simulink model "modelo_nioc_obs"  (R2023a)
settings: Solver=ode15s  StartTime=0.0  StopTime=100  RelTol=1e-3
InitFcn:
  | clc
  | clear
  | close all
  | parametros
  | gain_CL
  | calculo_observador_carro
  | calculo_observador_izaje
values from neighbouring files (symbols this model uses):
  At = [ 0, 1, 0, 0 ... (first row only)    [calculo_observador_carro.m]
  b_cx = 1e6    (= 1000000)    [parametros.m]
  b_cy = 1e7    (= 10000000)    [parametros.m]
  b_ha = -(J_hEq + (r_hd/(2*i_h))*m_l) * w_des_h*(1 + n_h + n_h^2) + b_hEq    [gain_CL.m]
  b_hb = 1e8    (= 100000000)    [parametros.m]
  b_hd = 8    [parametros.m]
  b_hm = 18    [parametros.m]
  b_t = 90    [parametros.m]
  b_ta = M_tEq*w_des_t*(1+n_t+n_t^2)-b_tEq    [gain_CL.m]
  b_tb = 5e6    (= 5000000)    [parametros.m]
  b_td = 1.8    [parametros.m]
  b_tm = 6    [parametros.m]
  b_tw = 3e3    (= 3000)    [parametros.m]
  b_wu = 150    [parametros.m]
  Bct = [ 0, 0 ... (first row only)    [calculo_observador_carro.m]
  Bdt = [ 0 ... (first row only)    [calculo_observador_carro.m]
  Ct = [ 1, 0, 0, 0 ]    [calculo_observador_carro.m]
  g = 9.80665    [parametros.m]
  H_c = 2.59    [parametros.m]
  i_h = 22    [parametros.m]
  i_t = 30    [parametros.m]
  J_hd_hEb = 3800    [parametros.m]
  J_hm_hb = 30    [parametros.m]
  J_td = 1200    [parametros.m]
  J_tm_tb = 7    [parametros.m]
  K_cy = 1.8e9    (= 1800000000)    [parametros.m]
  k_hsa = -(J_hEq + (r_hd/(2*i_h))*m_l) * w_des_h^2*(n_h + n_h^2 + n_h^3)    [gain_CL.m]
  k_hsia = -(J_hEq + (r_hd/(2*i_h))*m_l) * n_h^3 * w_des_h^3    [gain_CL.m]
  k_tsa = M_tEq*w_des_t^2*n_t*(1+n_t+n_t^2)    [gain_CL.m]
  k_tsia = M_tEq*w_des_t^3*n_t^3    [gain_CL.m]
  K_tw = 4.8e5    (= 480000)    [parametros.m]
  k_wu = 2.36e8    (= 236000000)    [parametros.m]
  l_h0 = (Y_t0-y_l0)    (= 38)    [parametros.m]
  Lt = place(At', Ct', polos_deseados)'    [calculo_observador_carro.m]
  M_cmax = 50000    [parametros.m]
  M_cmin = 2000    [parametros.m]
  m_l = M_s    (= 15000)    [parametros.m]
  M_s = 15000    [parametros.m]
  M_t = 30000    [parametros.m]
  M_tEq = i_t/r_td*(J_tm_tb+J_td/i_t^2)+r_td/i_t*(M_t+m_l)    (= 1250)    [parametros.m]
  r_hd = 0.75    [parametros.m]
  r_td = 0.50    (= 0.5)    [parametros.m]
  T_hbMax = 5e4    (= 50000)    [parametros.m]
  T_hEbMax = 1.1e6    (= 1100000)    [parametros.m]
  T_hmMax = 2e4    (= 20000)    [parametros.m]
  T_s = 0.001    [parametros.m]
  T_tbMax = 5e3    (= 5000)    [parametros.m]
  T_tmMax = 4e3    (= 4000)    [parametros.m]
  tau_tm = 1e-3    (= 0.001)    [parametros.m]
  theta_hm0 = -l_h0*i_h*2/r_hd    (= -2229.33333333)    [parametros.m]
  theta_tm0 = (x_t0)*i_t/r_td    (= -900)    [parametros.m]
  v_h_max_noload = 3    [parametros.m]
  v_lx0 = 0    [parametros.m]
  v_ly0 = 0    [parametros.m]
  v_t0 = 0    [parametros.m]
  v_t_max = 4    [parametros.m]
  W_c = ctrb(A, B_c(:,1))    [CyO_carro.m]    (also in CyO_izaje.m; parametros.m = 2.44)
  w_hm0 = 0    [parametros.m]
  w_hm_rated = v_h_max_load*2*i_h/r_hd    (= 88)    [parametros.m]
  w_tm0 = (v_t0)*i_t/r_td    (= 0)    [parametros.m]
  x_l0 = x_t0    (= -15)    [parametros.m]
  x_lidar_offset = 3.0    (= 3)    [parametros.m]
  x_t0 = -15    [parametros.m]
  x_t_max = 50    [parametros.m]
  x_t_maxE = x_t_max+0.5    (= 50.5)    [parametros.m]
  x_t_min = -30    [parametros.m]
  x_t_minE = x_t_min-0.5    (= -30.5)    [parametros.m]
  y_h_max = 40    [parametros.m]
  y_h_maxE = y_h_max+0.5    (= 40.5)    [parametros.m]
  y_h_min = -20    [parametros.m]
  y_h_minE = y_h_min-0.5    (= -20.5)    [parametros.m]
  y_l0 = 7    [parametros.m]
  Y_sb = 5.0    (= 5)    [parametros.m]
  Y_t0 = 45    [parametros.m]
undefined symbols (not defined in the file or in its folder): Lh
libraries: dspsigops x1, simulink x1
settings Model: Creator=Usuario  LastModifiedBy=nsorr

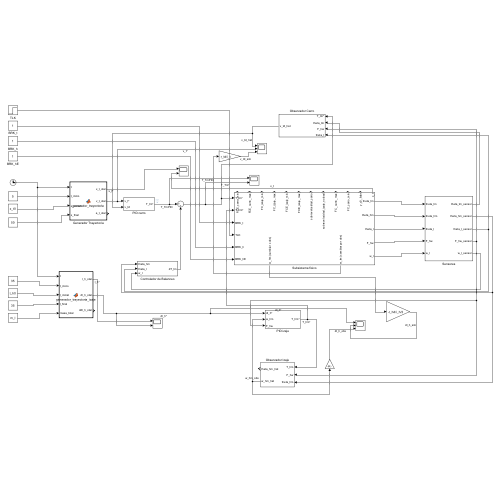
[thumbnail: Simulink's stored preview of the top-level diagram]
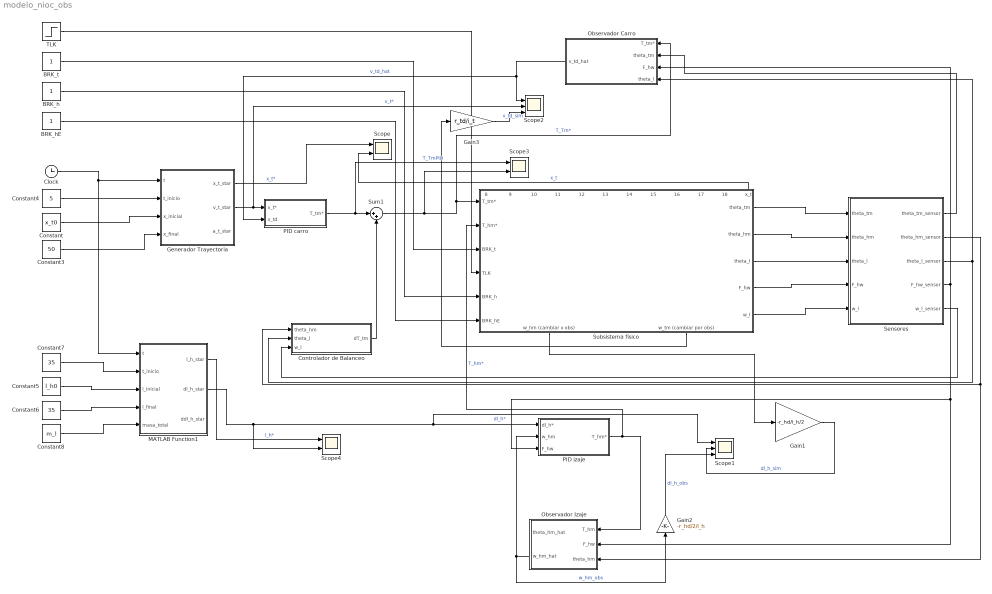
== system modelo_nioc_obs ==
  BRK_h : Constant
  BRK_hE : Constant
  BRK_t : Constant
  Clock : Clock
  Constant : Constant  Value=x_t0
  Constant3 : Constant  Value=50
  Constant4 : Constant  Value=5
  Constant5 : Constant  Value=l_h0
  Constant6 : Constant  Value=35
  Constant7 : Constant  Value=35
  Constant8 : Constant  Value=m_l
  Controlador de Balanceo : Subsystem
  Gain1 : Gain  Gain=-r_hd/i_h/2
  Gain2 : Gain  Gain=-r_hd/2/i_h
  Gain3 : Gain  Gain=r_td/i_t
  Generador Trayectoria : MATLAB Function  TreatAsAtomicUnit=on
  MATLAB Function1 : MATLAB Function  TreatAsAtomicUnit=on
  Observador Carro : Subsystem
  Observador Izaje : Subsystem
  PID carro : Subsystem
  PID izaje : Subsystem
  Scope : Scope  NumInputPorts=2
  Scope1 : Scope  NumInputPorts=3
  Scope2 : Scope  NumInputPorts=3
  Scope3 : Scope  NumInputPorts=2
  Scope4 : Scope  NumInputPorts=2
  Sensores : Subsystem
  Subsistema físico : Subsystem
      settings: PortSchema="{\"entries\":[{\"content\":{\"sides\":[{\"content\":{\"connectorIds\":[\"In1\",\"In2\",\"In3\",\"In4\",\"In5\",\"In6\"]},\"type\":\"ConnectorPlacement.EquallySpacedRectSide\",\"uuid\":\"aa1cb789-2051-45a4-8cb8-6dd2078290cc\"},{\"content\":{\"connectorIds\":[\"Out1\",\"Out2\",\"Out3\",\"Out4\",\"Out5\"],\"side\":\"RIGHT\"},\"type\":\"ConnectorPlacement.EquallySpacedRectSide\",\"uuid\":\"7fe62279-dd3b-46db-ba9e-e4633dcea5c6\"},{\"content\":{\"connectorIds\":[\"Out8\",\"Out9\",\"Out10\",\"Out11\",\"Out12\",\"Out13\",\"Out14\",\"Out15\",\"Out16\",\"Out17\",\"Out18\",\"Out19\"],\"side\":\"TOP\"},\"type\":\"ConnectorPlacement.EquallySpacedRectSide\",\"uuid\":\"a5663ea7-10d8-47d7-b8ed-8fbfb239b85a\"},{\"content\":{\"connectorIds\":[\"Out6\",\"Out7\"],\"side\":\"BOTTOM\"},\"type\":\"ConnectorPlacement.EquallySpacedRectSide\",\"uuid\":\"9ec9131f-7b2f-42d7-8a86-9462c3c282b3\"}]},\"type\":\"ConnectorPlacement.EquallySpacedConnector\",\"uuid\":\"e7df1a56-7803-4e0d-8bf9-081877eb8c08\"}],\"packageUris\":[\"http://schema.mathworks.com/mf0/Connector/R2020b\"],\"version\":\"1.0\"}"
  Sum1 : Sum  Inputs=|++
  TLK : Step  Time=5  SampleTime=0
  wires:
  Constant8/1 -> MATLAB Function1/5(masa_total)
  Generador Trayectoria/2(v_t_star) -> Scope2/2, PID carro/1(v_t*)  "v_t*"
  Constant7/1 -> MATLAB Function1/2(t_inicio)
  BRK_h/1 -> Subsistema físico/5(BRK_h)
  Constant6/1 -> MATLAB Function1/4(l_final)
  PID carro/1(T_tm*) -> Scope3/1, Sum1/1  "T_TmPID"
  BRK_t/1 -> Subsistema físico/3(BRK_t)
  Subsistema físico/2(theta_hm) -> Sensores/2(theta_hm)
  Constant4/1 -> Generador Trayectoria/2(t_inicio)
  Constant5/1 -> MATLAB Function1/3(l_inicial)
  MATLAB Function1/2(dl_h_star) -> Scope4/2, Scope1/1, PID izaje/1(dl_h*)  "dl_h*"
  BRK_hE/1 -> Subsistema físico/6(BRK_hE)
  Constant3/1 -> Generador Trayectoria/4(x_final)
  Subsistema físico/1(theta_tm) -> Sensores/1(theta_tm)
  Clock/1 -> MATLAB Function1/1(t), Generador Trayectoria/1(t)
  Constant/1 -> Generador Trayectoria/3(x_inicial)
  TLK/1 -> Subsistema físico/4(TLK)
  Subsistema físico/3(theta_l) -> Sensores/3(theta_l)
  Controlador de Balanceo/1(dT_tm) -> Sum1/2
  Subsistema físico/4(F_hw) -> Sensores/4(F_hw)
  Subsistema físico/5(w_l) -> Sensores/5(w_l)
  Sensores/3(theta_l_sensor) -> Observador Carro/4(theta_l), Controlador de Balanceo/2(theta_l)
  Sensores/4(F_hw_sensor) -> Observador Carro/3(F_hw), Observador Izaje/2(F_hw), PID izaje/3(F_hw)
  Sensores/2(theta_hm_sensor) -> Observador Izaje/3(theta_hm), Controlador de Balanceo/1(theta_hm)
  Sensores/5(w_l_sensor) -> Controlador de Balanceo/3(w_l)
  PID izaje/1(T_hm*) -> Observador Izaje/1(T_hm), Subsistema físico/2(T_hm*)  "T_hm*"
  Gain1/1 -> Scope1/2  "dl_h_sim"
  Sum1/1 -> Scope3/2, Observador Carro/1(T_tm*), Subsistema físico/1(T_tm*)  "T_Tm*"
  Observador Izaje/2(w_hm_hat) -> PID izaje/2(w_hm), Gain2/1  "w_hm_obs"
  Gain2/1 -> Scope1/3  "dl_h_obs"
  Subsistema físico/6(w_hm (cambiar x obs)) -> Gain1/1
  Sensores/1(theta_tm_sensor) -> Observador Carro/2(theta_tm)
  Observador Carro/1(v_td_hat) -> PID carro/2(v_td), Scope2/1  "v_td_hat"
  Gain3/1 -> Scope2/3  "v_td_sim"
  Subsistema físico/7(w_tm (cambiar por obs)) -> Gain3/1
  Generador Trayectoria/1(x_t_star) -> Scope/1  "x_t*"
  Subsistema físico/19(x_t) -> Scope/2  "x_t"
  MATLAB Function1/1(l_h_star) -> Scope4/1  "l_h*"

== system modelo_nioc_obs/Controlador de Balanceo ==
  theta_hm : Inport
  theta_l : Inport  Port=2
  w_l : Inport  Port=3
  Constant1 : Constant  Value=g
  Derivative1 : Derivative
  Gain2 : Gain  Gain=M_tEq * r_td / i_t
  Gain3 : Gain  Gain=r_hd/i_h/2
  MATLAB Function : MATLAB Function  TreatAsAtomicUnit=on
  dT_tm : Outport
  wires:
  Gain3/1 -> Derivative1/1, MATLAB Function/3(l)
  Derivative1/1 -> MATLAB Function/4(dl_dt)
  theta_l/1 -> MATLAB Function/1(theta_l)
  Constant1/1 -> MATLAB Function/5(g)
  MATLAB Function/1(a_PD) -> Gain2/1
  theta_hm/1 -> Gain3/1
  Gain2/1 -> dT_tm/1
  w_l/1 -> MATLAB Function/2(w_l)

== system modelo_nioc_obs/Observador Carro ==
  T_tm* : Inport
  theta_tm : Inport  Port=2
  F_hw : Inport  Port=3
  theta_l : Inport  Port=4
  Constant : Constant  Value=0
  Gain : Gain  Gain=r_td/i_t
  Mux : Mux
  Product : Product
  Sin : Trigonometry
  State-Space : StateSpace  A=At-Lt*Ct  B=[Bct, Bdt, Lt]  C=[0 1 0 0]  D=[0 0 0 0]  InitialCondition=[theta_tm0, 0, x_t0, 0]
  v_td_hat : Outport
  wires:
  theta_l/1 -> Sin/1
  F_hw/1 -> Product/1
  Sin/1 -> Product/2
  Product/1 -> Mux/3
  theta_tm/1 -> Mux/4
  T_tm*/1 -> Mux/1
  Constant/1 -> Mux/2
  Mux/1 -> State-Space/1
  State-Space/1 -> Gain/1
  Gain/1 -> v_td_hat/1

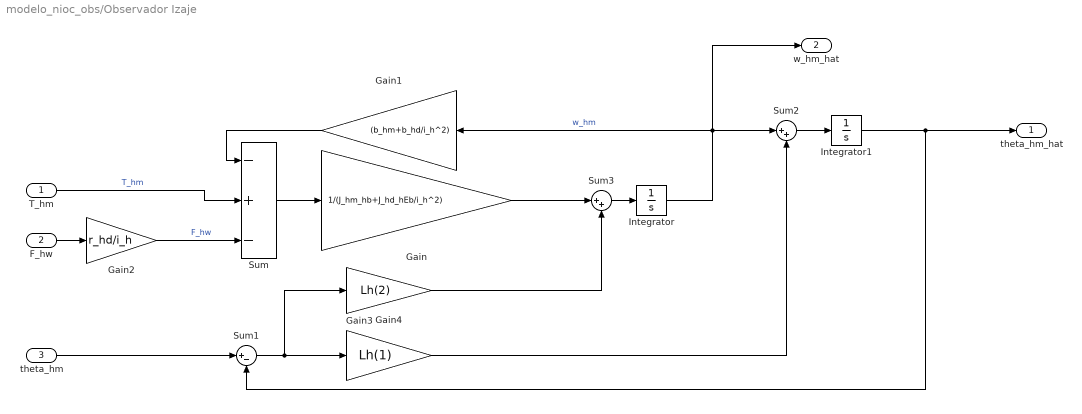
== system modelo_nioc_obs/Observador Izaje ==
  T_hm : Inport
  F_hw : Inport  Port=2
  theta_hm : Inport  Port=3
  Gain : Gain  Gain=1/(J_hm_hb+J_hd_hEb/i_h^2)
  Gain1 : Gain  Gain=(b_hm+b_hd/i_h^2)
  Gain2 : Gain  Gain=r_hd/i_h
  Gain3 : Gain  Gain=Lh(1)
  Gain4 : Gain  Gain=Lh(2)
  Integrator : Integrator
  Integrator1 : Integrator  InitialCondition=theta_hm0
  Sum : Sum  Inputs=-+-
  Sum1 : Sum  Inputs=|+-
  Sum2 : Sum  Inputs=|++
  Sum3 : Sum  Inputs=|++
  theta_hm_hat : Outport
  w_hm_hat : Outport  Port=2
  wires:
  F_hw/1 -> Gain2/1
  Gain1/1 -> Sum/1
  Gain/1 -> Sum3/1
  Sum/1 -> Gain/1
  T_hm/1 -> Sum/2  "T_hm"
  Integrator/1 -> Sum2/1, w_hm_hat/1, Gain1/1  "w_hm"
  Integrator1/1 -> Sum1/2, theta_hm_hat/1
  Gain2/1 -> Sum/3  "F_hw"
  theta_hm/1 -> Sum1/1
  Sum1/1 -> Gain4/1, Gain3/1
  Gain3/1 -> Sum2/2
  Sum2/1 -> Integrator1/1
  Sum3/1 -> Integrator/1
  Gain4/1 -> Sum3/2

== system modelo_nioc_obs/PID carro ==
  v_t* : Inport
  v_td : Inport  Port=2
  Gain : Gain  Gain=b_ta
  Gain1 : Gain  Gain=k_tsia
  Gain2 : Gain  Gain=k_tsa
  Integrator : Integrator  LimitOutput=on  UpperSaturationLimit=4e3  LowerSaturationLimit=-4e3
  Integrator1 : Integrator  LimitOutput=on  UpperSaturationLimit=4e3  LowerSaturationLimit=-4e3
  Sum : Sum  Inputs=|+-
  Sum1 : Sum  Inputs=+++
  T_tm* : Outport
  wires:
  Gain2/1 -> Sum1/2  "P"
  v_t*/1 -> Sum/1
  Gain/1 -> Sum1/3  "D"
  Gain1/1 -> Sum1/1  "I"
  Sum1/1 -> T_tm*/1
  Sum/1 -> Integrator1/1, Gain/1  "e"
  Integrator1/1 -> Integrator/1, Gain2/1
  Integrator/1 -> Gain1/1
  v_td/1 -> Sum/2

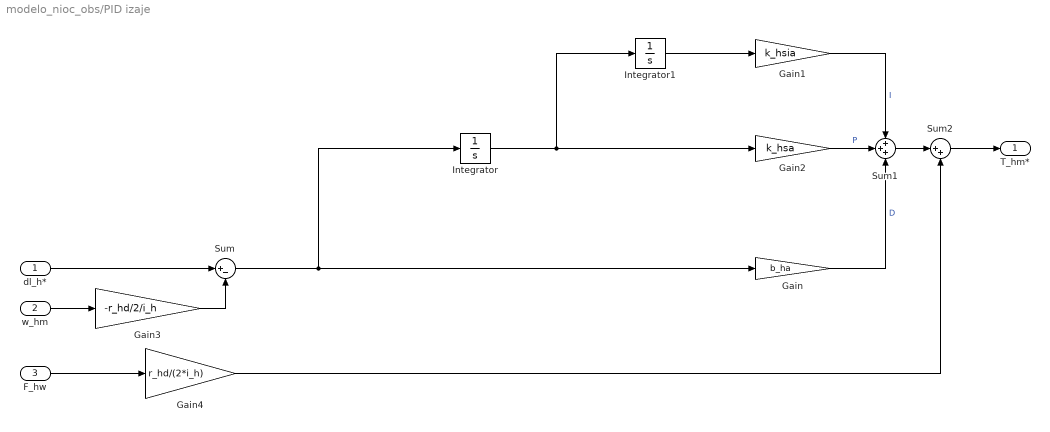
== system modelo_nioc_obs/PID izaje ==
  dl_h* : Inport
  w_hm : Inport  Port=2
  F_hw : Inport  Port=3
  Gain : Gain  Gain=b_ha
  Gain1 : Gain  Gain=k_hsia
  Gain2 : Gain  Gain=k_hsa
  Gain3 : Gain  Gain=-r_hd/2/i_h
  Gain4 : Gain  Gain=r_hd/(2*i_h)
  Integrator : Integrator
  Integrator1 : Integrator
  Sum : Sum  Inputs=|+-
  Sum1 : Sum  Inputs=+++
  Sum2 : Sum  Inputs=|++
  T_hm* : Outport
  wires:
  Gain2/1 -> Sum1/2  "P"
  dl_h*/1 -> Sum/1
  Gain/1 -> Sum1/3  "D"
  Gain1/1 -> Sum1/1  "I"
  w_hm/1 -> Gain3/1
  Sum1/1 -> Sum2/1
  Sum/1 -> Integrator/1, Gain/1
  Integrator/1 -> Integrator1/1, Gain2/1
  Integrator1/1 -> Gain1/1
  Gain3/1 -> Sum/2
  Sum2/1 -> T_hm*/1
  Gain4/1 -> Sum2/2
  F_hw/1 -> Gain4/1

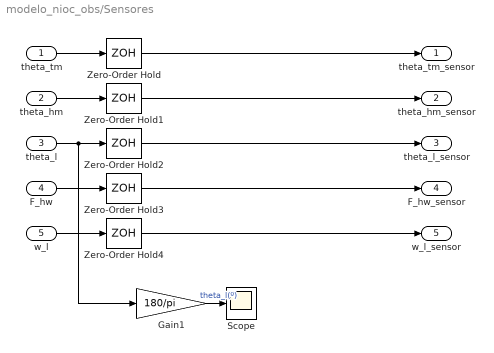
== system modelo_nioc_obs/Sensores ==
  theta_tm : Inport
  theta_hm : Inport  Port=2
  theta_l : Inport  Port=3
  F_hw : Inport  Port=4
  w_l : Inport  Port=5
  Gain1 : Gain  Gain=180/pi
  Scope : Scope
  Zero-Order Hold{,1..4} (5 alike) : ZeroOrderHold  SampleTime=T_s
  theta_tm_sensor : Outport
  theta_hm_sensor : Outport  Port=2
  theta_l_sensor : Outport  Port=3
  F_hw_sensor : Outport  Port=4
  w_l_sensor : Outport  Port=5
  wires:
  theta_tm/1 -> Zero-Order Hold/1
  Zero-Order Hold/1 -> theta_tm_sensor/1
  Zero-Order Hold1/1 -> theta_hm_sensor/1
  theta_hm/1 -> Zero-Order Hold1/1
  w_l/1 -> Zero-Order Hold4/1
  F_hw/1 -> Zero-Order Hold3/1
  theta_l/1 -> Gain1/1, Zero-Order Hold2/1
  Zero-Order Hold2/1 -> theta_l_sensor/1
  Zero-Order Hold3/1 -> F_hw_sensor/1
  Zero-Order Hold4/1 -> w_l_sensor/1
  Gain1/1 -> Scope/1  "theta_l(º)"

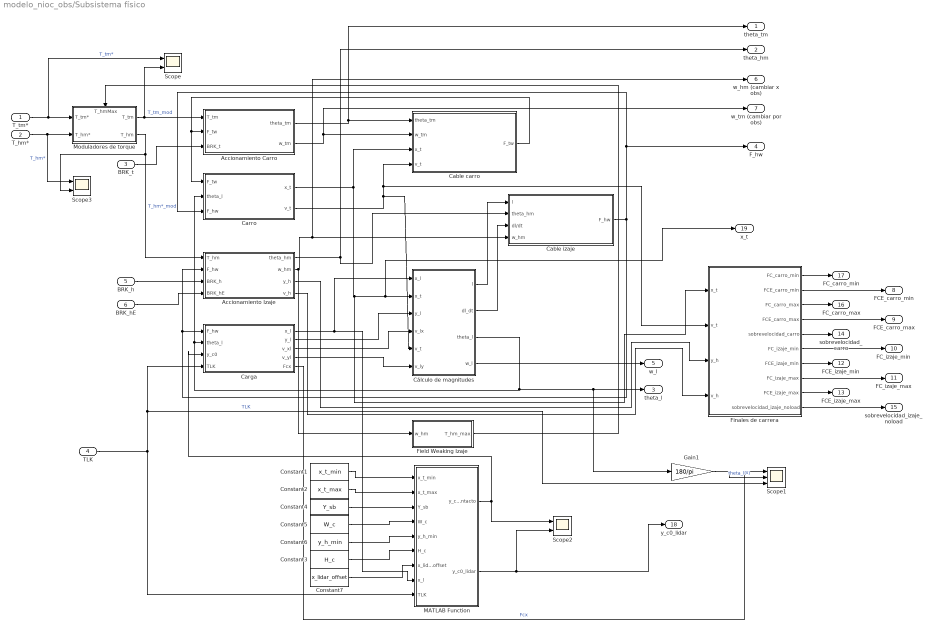
== system modelo_nioc_obs/Subsistema físico ==
  T_tm* : Inport
  T_hm* : Inport  Port=2
  BRK_t : Inport  Port=3
  TLK : Inport  Port=4
  BRK_h : Inport  Port=5
  BRK_hE : Inport  Port=6
  Accionamiento Carro : Subsystem
  Accionamiento Izaje : Subsystem
  Cable carro : Subsystem
  Cable izaje : Subsystem
  Carga : Subsystem
  Carro : Subsystem
  Constant1 : Constant  Value=x_t_min
  Constant2 : Constant  Value=x_t_max
  Constant3 : Constant  Value=H_c
  Constant4 : Constant  Value=Y_sb
  Constant5 : Constant  Value=W_c
  Constant6 : Constant  Value=y_h_min
  Constant7 : Constant  Value=x_lidar_offset
  Cálculo de magnitudes : Subsystem
  Field Weaking Izaje : Subsystem
  Finales de carrera : Subsystem
  Gain1 : Gain  Gain=180/pi
  MATLAB Function : MATLAB Function  TreatAsAtomicUnit=on  SystemSampleTime=T_s
  Moduladores de torque : Subsystem
      settings: PortSchema="{\"entries\":[{\"content\":{\"sides\":[{\"content\":{\"connectorIds\":[\"In1\",\"In2\"]},\"type\":\"ConnectorPlacement.EquallySpacedRectSide\",\"uuid\":\"c66d3892-523c-433a-8dde-517eb495bac1\"},{\"content\":{\"connectorIds\":[\"Out1\",\"Out2\"],\"side\":\"RIGHT\"},\"type\":\"ConnectorPlacement.EquallySpacedRectSide\",\"uuid\":\"bbb0a9b0-6ff9-4fa8-ace8-11da5b7abadd\"},{\"content\":{\"connectorIds\":[\"In3\"],\"side\":\"TOP\"},\"type\":\"ConnectorPlacement.EquallySpacedRectSide\",\"uuid\":\"35baaaad-8e6c-401a-84f7-749de5492b29\"}]},\"type\":\"ConnectorPlacement.EquallySpacedConnector\",\"uuid\":\"d8d05b6c-004b-40f1-854a-ea077232777a\"}],\"packageUris\":[\"http://schema.mathworks.com/mf0/Connector/R2020b\"],\"version\":\"1.0\"}"
  Scope : Scope  NumInputPorts=2
  Scope1 : Scope  NumInputPorts=3
  Scope2 : Scope  NumInputPorts=2
  Scope3 : Scope  NumInputPorts=2
  theta_tm : Outport
  theta_hm : Outport  Port=2
  theta_l : Outport  Port=3
  F_hw : Outport  Port=4
  w_l : Outport  Port=5
  w_hm (cambiar x obs) : Outport  Port=6
  w_tm (cambiar por obs) : Outport  Port=7
  FCE_carro_min : Outport  Port=8
  FCE_carro_max : Outport  Port=9
  FC_izaje_min : Outport  Port=10
  FC_izaje_max : Outport  Port=11
  FCE_izaje_min : Outport  Port=12
  FCE_izaje_max : Outport  Port=13
  sobrevelocidad_carro : Outport  Port=14
  sobrevelocidad_izaje_noload : Outport  Port=15
  FC_carro_max : Outport  Port=16
  FC_carro_min : Outport  Port=17
  y_c0_lidar : Outport  Port=18
  x_t : Outport  Port=19
  wires:
  T_tm*/1 -> Scope/1, Moduladores de torque/1(T_tm*)  "T_tm*"
  Accionamiento Carro/1(theta_tm) -> theta_tm/1, Cable carro/1(theta_tm)
  Accionamiento Carro/2(w_tm) -> w_tm (cambiar por obs)/1, Cable carro/2(w_tm)
  Carro/1(x_t) -> Finales de carrera/1(x_t), x_t/1, Cálculo de magnitudes/2(x_t), Cable carro/3(x_t)
  Carro/2(v_t) -> Cálculo de magnitudes/5(v_t), Cable carro/4(v_t), Finales de carrera/2(v_t)
  Cable carro/1(F_tw) -> Carro/1(F_tw), Accionamiento Carro/2(F_tw)
  Carga/1(x_l) -> MATLAB Function/8(x_l), Cálculo de magnitudes/1(x_l)
  Carga/2(y_l) -> Cálculo de magnitudes/3(y_l)
  Carga/3(v_xl) -> Cálculo de magnitudes/4(v_lx)
  Carga/4(v_yl) -> Cálculo de magnitudes/6(v_ly)
  Cálculo de magnitudes/1(l) -> Cable izaje/1(l)
  Accionamiento Izaje/1(theta_hm) -> Cable izaje/2(theta_hm), theta_hm/1
  Cable izaje/1(F_hw) -> F_hw/1, Carro/3(F_hw), Accionamiento Izaje/2(F_hw), Carga/1(F_hw)
  Cálculo de magnitudes/2(dl_dt) -> Cable izaje/3(dl/dt)
  T_hm*/1 -> Scope3/1, Moduladores de torque/2(T_hm*)  "T_hm*"
  Accionamiento Izaje/2(w_hm) -> Field Weaking Izaje/1(w_hm), w_hm (cambiar x obs)/1, Cable izaje/4(w_hm)
  Cálculo de magnitudes/3(theta_l) -> Carro/2(theta_l), Carga/2(theta_l), Gain1/1, theta_l/1
  BRK_t/1 -> Accionamiento Carro/3(BRK_t)
  BRK_h/1 -> Accionamiento Izaje/3(BRK_h)
  BRK_hE/1 -> Accionamiento Izaje/4(BRK_hE)
  TLK/1 -> Scope1/3, Carga/4(TLK), MATLAB Function/9(TLK)  "TLK"
  Accionamiento Izaje/3(y_h) -> Finales de carrera/3(y_h)
  Accionamiento Izaje/4(v_h) -> Finales de carrera/4(v_h)
  Cálculo de magnitudes/4(w_l) -> w_l/1
  Moduladores de torque/1(T_tm) -> Scope/2, Accionamiento Carro/1(T_tm)  "T_tm_mod"
  Field Weaking Izaje/1(T_hm_max) -> Moduladores de torque/3(T_hmMax)
  Moduladores de torque/2(T_hm) -> Scope3/2, Accionamiento Izaje/1(T_hm)  "T_hm*_mod"
  Finales de carrera/1(FC_carro_min) -> FC_carro_min/1
  Finales de carrera/2(FCE_carro_min) -> FCE_carro_min/1
  Finales de carrera/3(FC_carro_max) -> FC_carro_max/1
  Finales de carrera/4(FCE_carro_max) -> FCE_carro_max/1
  Finales de carrera/5(sobrevelocidad_carro) -> sobrevelocidad_carro/1
  Finales de carrera/7(FCE_izaje_min) -> FCE_izaje_min/1
  Finales de carrera/6(FC_izaje_min) -> FC_izaje_min/1
  Finales de carrera/8(FC_izaje_max) -> FC_izaje_max/1
  Finales de carrera/9(FCE_izaje_max) -> FCE_izaje_max/1
  Finales de carrera/10(sobrevelocidad_izaje_noload) -> sobrevelocidad_izaje_noload/1
  Constant1/1 -> MATLAB Function/1(x_t_min)
  Constant2/1 -> MATLAB Function/2(x_t_max)
  Constant3/1 -> MATLAB Function/6(H_c)
  Constant4/1 -> MATLAB Function/3(Y_sb)
  Constant5/1 -> MATLAB Function/4(W_c)
  Constant6/1 -> MATLAB Function/5(y_h_min)
  MATLAB Function/1(y_c0_contacto) -> Carga/3(y_c0), Scope2/1
  Constant7/1 -> MATLAB Function/7(x_lidar_offset)
  MATLAB Function/2(y_c0_lidar) -> Scope2/2, y_c0_lidar/1
  Carga/5(Fcx) -> Scope1/1  "Fcx"
  Gain1/1 -> Scope1/2  "theta_l(º)"

== system modelo_nioc_obs/Subsistema físico/Accionamiento Carro ==
  T_tm : Inport
  F_tw : Inport  Port=2
  BRK_t : Inport  Port=3
  Gain : Gain  Gain=1/(J_tm_tb+J_td/i_t^2)
  Gain1 : Gain  Gain=r_td/i_t
  Gain2 : Gain  Gain=(b_tm+b_td/i_t^2)
  Integrator : Integrator  InitialCondition=w_tm0
  Integrator1 : Integrator  InitialCondition=theta_tm0
  Subsystem : Subsystem
  Sum : Sum  Inputs=+-+-
  theta_tm : Outport
  w_tm : Outport  Port=2
  wires:
  Integrator1/1 -> theta_tm/1
  Integrator/1 -> w_tm/1, Gain2/1, Subsystem/2(w_tm), Integrator1/1  "w_tm"
  Gain/1 -> Integrator/1
  Sum/1 -> Gain/1
  T_tm/1 -> Sum/1
  F_tw/1 -> Gain1/1
  Gain1/1 -> Sum/2
  Subsystem/1(T_tb) -> Sum/3
  Gain2/1 -> Sum/4
  BRK_t/1 -> Subsystem/1(BRK_t)

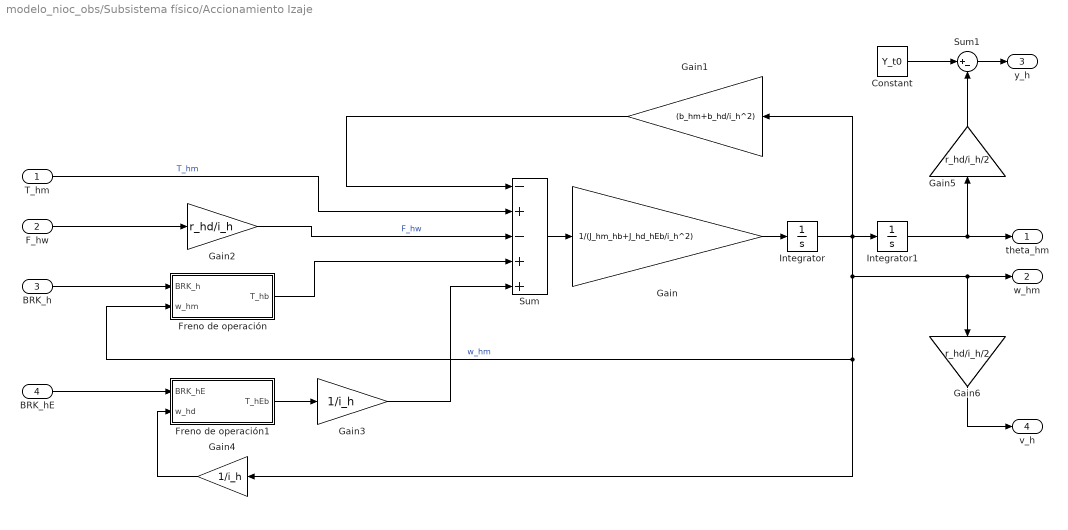
== system modelo_nioc_obs/Subsistema físico/Accionamiento Izaje ==
  T_hm : Inport
  F_hw : Inport  Port=2
  BRK_h : Inport  Port=3
  BRK_hE : Inport  Port=4
  Constant : Constant  Value=Y_t0
  Freno de operación : Subsystem
  Freno de operación1 : Subsystem
  Gain : Gain  Gain=1/(J_hm_hb+J_hd_hEb/i_h^2)
  Gain1 : Gain  Gain=(b_hm+b_hd/i_h^2)
  Gain2 : Gain  Gain=r_hd/i_h
  Gain3 : Gain  Gain=1/i_h
  Gain4 : Gain  Gain=1/i_h
  Gain5 : Gain  Gain=r_hd/i_h/2
  Gain6 : Gain  Gain=r_hd/i_h/2
  Integrator : Integrator  InitialCondition=w_hm0
  Integrator1 : Integrator  InitialCondition=theta_hm0
  Sum : Sum  Inputs=-+-++
  Sum1 : Sum  Inputs=|+-
  theta_hm : Outport
  w_hm : Outport  Port=2
  y_h : Outport  Port=3
  v_h : Outport  Port=4
  wires:
  Integrator1/1 -> Gain5/1, theta_hm/1
  Integrator/1 -> Integrator1/1, Gain6/1, w_hm/1, Gain4/1, Freno de operación/2(w_hm), Gain1/1  "w_hm"
  Gain/1 -> Integrator/1
  Sum/1 -> Gain/1
  Gain1/1 -> Sum/1
  F_hw/1 -> Gain2/1
  Gain2/1 -> Sum/3  "F_hw"
  T_hm/1 -> Sum/2  "T_hm"
  Freno de operación/1(T_hb) -> Sum/4
  BRK_h/1 -> Freno de operación/1(BRK_h)
  Freno de operación1/1(T_hEb) -> Gain3/1
  Gain3/1 -> Sum/5
  BRK_hE/1 -> Freno de operación1/1(BRK_hE)
  Gain4/1 -> Freno de operación1/2(w_hd)
  Sum1/1 -> y_h/1
  Gain5/1 -> Sum1/2
  Constant/1 -> Sum1/1
  Gain6/1 -> v_h/1

== system modelo_nioc_obs/Subsistema físico/Cable carro ==
  theta_tm : Inport
  w_tm : Inport  Port=2
  x_t : Inport  Port=3
  v_t : Inport  Port=4
  Gain : Gain  Gain=b_tw
  Gain1 : Gain  Gain=K_tw
  Gain2 : Gain  Gain=r_td/i_t
  Gain3 : Gain  Gain=r_td/i_t
  Sum : Sum  Inputs=|+-
  Sum1 : Sum  Inputs=|+-
  Sum2 : Sum  Inputs=|++
  F_tw : Outport
  wires:
  Sum/1 -> Gain1/1
  theta_tm/1 -> Gain3/1
  x_t/1 -> Sum/2
  Sum1/1 -> Gain/1
  w_tm/1 -> Gain2/1
  v_t/1 -> Sum1/2
  Gain/1 -> Sum2/2
  Gain1/1 -> Sum2/1
  Sum2/1 -> F_tw/1
  Gain2/1 -> Sum1/1  "v_td"
  Gain3/1 -> Sum/1  "x_td"

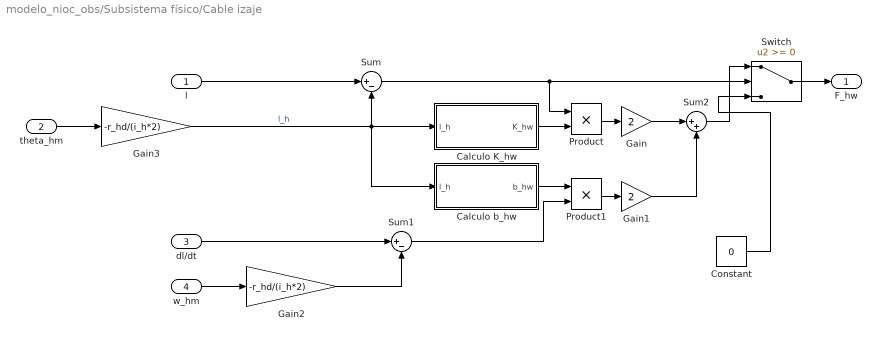
== system modelo_nioc_obs/Subsistema físico/Cable izaje ==
  l : Inport
  theta_hm : Inport  Port=2
  dl/dt : Inport  Port=3
  w_hm : Inport  Port=4
  Calculo K_hw : Subsystem
  Calculo b_hw : Subsystem
  Constant : Constant  Value=0
  Gain : Gain  Gain=2
  Gain1 : Gain  Gain=2
  Gain2 : Gain  Gain=-r_hd/(i_h*2)
  Gain3 : Gain  Gain=-r_hd/(i_h*2)
  Product : Product
  Product1 : Product
  Sum : Sum  Inputs=|+-
  Sum1 : Sum  Inputs=|+-
  Sum2 : Sum  Inputs=|++
  Switch : Switch  SaturateOnIntegerOverflow=off  InputSameDT=off
  F_hw : Outport
  wires:
  l/1 -> Sum/1
  theta_hm/1 -> Gain3/1
  Sum/1 -> Product/1, Switch/2
  Calculo K_hw/1(K_hw) -> Product/2
  Product/1 -> Gain/1
  w_hm/1 -> Gain2/1
  Product1/1 -> Gain1/1
  Calculo b_hw/1(b_hw) -> Product1/1
  Gain1/1 -> Sum2/2
  Gain/1 -> Sum2/1
  Sum2/1 -> Switch/1
  Switch/1 -> F_hw/1
  dl/dt/1 -> Sum1/1
  Constant/1 -> Switch/3
  Gain2/1 -> Sum1/2
  Gain3/1 -> Calculo b_hw/1(l_h), Calculo K_hw/1(l_h), Sum/2  "l_h"
  Sum1/1 -> Product1/2

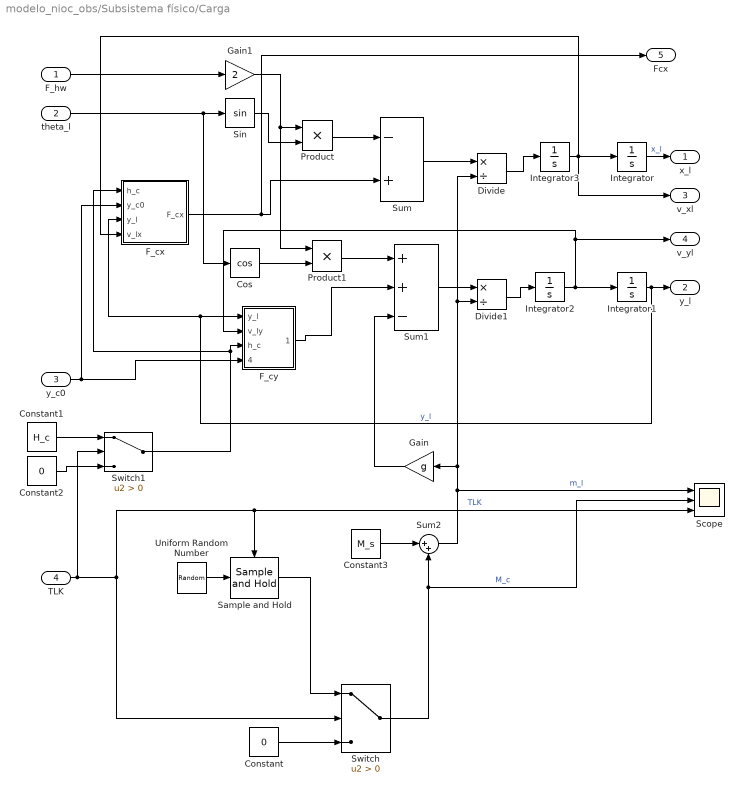
== system modelo_nioc_obs/Subsistema físico/Carga ==
  F_hw : Inport
  theta_l : Inport  Port=2
  y_c0 : Inport  Port=3
  TLK : Inport  Port=4
  Constant : Constant  Value=0
  Constant1 : Constant  Value=H_c
  Constant2 : Constant  Value=0
  Constant3 : Constant  Value=M_s
  Cos : Trigonometry  Operator=cos
  Divide : Product  Inputs=*/
  Divide1 : Product  Inputs=*/
  F_cx : Subsystem
  F_cy : Subsystem
  Gain : Gain  Gain=g
  Gain1 : Gain  Gain=2
  Integrator : Integrator  InitialCondition=x_l0
  Integrator1 : Integrator  InitialCondition=y_l0
  Integrator2 : Integrator  InitialCondition=v_ly0
  Integrator3 : Integrator  InitialCondition=v_lx0
  Product : Product
  Product1 : Product
  Sample and Hold : dspsigops/Sample and Hold  trig=Rising edge  initCond=0  latchinput=off
  Scope : Scope  NumInputPorts=3
  Sin : Trigonometry
  Sum : Sum  Inputs=-+
  Sum1 : Sum  Inputs=++-
  Sum2 : Sum  Inputs=|++
  Switch : Switch  Criteria=u2 > Threshold  SaturateOnIntegerOverflow=off  InputSameDT=off
  Switch1 : Switch  Criteria=u2 > Threshold  SaturateOnIntegerOverflow=off  InputSameDT=off
  Uniform Random Number : UniformRandomNumber  Minimum=M_cmin  Maximum=M_cmax  SampleTime=1
  x_l : Outport
  y_l : Outport  Port=2
  v_xl : Outport  Port=3
  v_yl : Outport  Port=4
  Fcx : Outport  Port=5
  wires:
  Sum/1 -> Divide/1
  Divide/1 -> Integrator3/1
  theta_l/1 -> Cos/1, Sin/1
  F_hw/1 -> Gain1/1
  Gain1/1 -> Product/1, Product1/1
  Sin/1 -> Product/2
  Product/1 -> Sum/1
  Switch1/1 -> F_cx/1(h_c), F_cy/3(h_c)
  Product1/1 -> Sum1/1
  Cos/1 -> Product1/2
  F_cy/1(F_cy) -> Sum1/2
  Divide1/1 -> Integrator2/1
  Sum1/1 -> Divide1/1
  Integrator/1 -> x_l/1  "x_l"
  Integrator3/1 -> v_xl/1, F_cx/4(v_lx), Integrator/1
  Integrator2/1 -> v_yl/1, F_cy/2(v_ly), Integrator1/1
  Integrator1/1 -> F_cx/3(y_l), F_cy/1(y_l), y_l/1  "y_l"
  y_c0/1 -> F_cx/2(y_c0), F_cy/4(y_c0)
  F_cx/1(F_cx) -> Fcx/1, Sum/2
  TLK/1 -> Switch1/2, Scope/3, Sample and Hold/Trigger, Switch/2  "TLK"
  Switch/1 -> Scope/2, Sum2/2  "M_c"
  Constant3/1 -> Sum2/1
  Sum2/1 -> Gain/1, Divide1/2, Divide/2, Scope/1  "m_l"
  Uniform Random Number/1 -> Sample and Hold/1
  Sample and Hold/1 -> Switch/1
  Constant/1 -> Switch/3
  Constant1/1 -> Switch1/1
  Constant2/1 -> Switch1/3
  Gain/1 -> Sum1/3

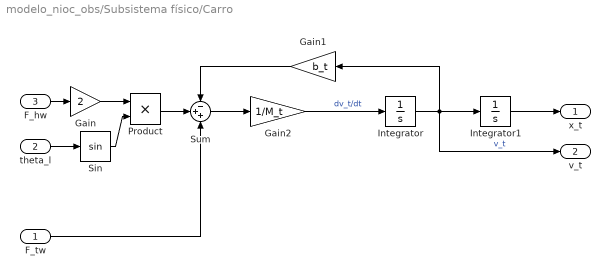
== system modelo_nioc_obs/Subsistema físico/Carro ==
  F_tw : Inport
  theta_l : Inport  Port=2
  F_hw : Inport  Port=3
  Gain : Gain  Gain=2
  Gain1 : Gain  Gain=b_t
  Gain2 : Gain  Gain=1/M_t
  Integrator : Integrator  InitialCondition=v_t0
  Integrator1 : Integrator  InitialCondition=x_t0
  Product : Product
  Sin : Trigonometry
  Sum : Sum  Inputs=-++
  x_t : Outport
  v_t : Outport  Port=2
  wires:
  F_tw/1 -> Sum/3
  F_hw/1 -> Gain/1
  Gain/1 -> Product/1
  theta_l/1 -> Sin/1
  Sin/1 -> Product/2
  Product/1 -> Sum/2
  Integrator/1 -> v_t/1, Integrator1/1, Gain1/1  "v_t"
  Sum/1 -> Gain2/1
  Gain2/1 -> Integrator/1  "dv_t/dt"
  Integrator1/1 -> x_t/1
  Gain1/1 -> Sum/1

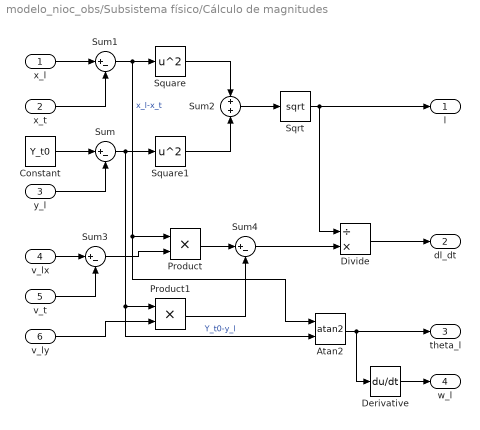
== system modelo_nioc_obs/Subsistema físico/Cálculo de magnitudes ==
  x_l : Inport
  x_t : Inport  Port=2
  y_l : Inport  Port=3
  v_lx : Inport  Port=4
  v_t : Inport  Port=5
  v_ly : Inport  Port=6
  Atan2 : Trigonometry  Operator=atan2
  Constant : Constant  Value=Y_t0
  Derivative : Derivative
  Divide : Product  Inputs=/*
  Product : Product
  Product1 : Product
  Sqrt : Sqrt
  Square : Math  Operator=square
  Square1 : Math  Operator=square
  Sum{,1,3..4} (4 alike) : Sum  Inputs=|+-
  Sum2 : Sum  Inputs=+|+
  l : Outport
  dl_dt : Outport  Port=2
  theta_l : Outport  Port=3
  w_l : Outport  Port=4
  wires:
  Constant/1 -> Sum/1
  y_l/1 -> Sum/2
  x_l/1 -> Sum1/1
  x_t/1 -> Sum1/2
  Sum1/1 -> Atan2/1, Product/1, Square/1  "x_l-x_t"
  Sum/1 -> Atan2/2, Product1/1, Square1/1  "Y_t0-y_l"
  Square/1 -> Sum2/1
  Square1/1 -> Sum2/2
  Sum2/1 -> Sqrt/1
  Sqrt/1 -> Divide/1, l/1
  v_lx/1 -> Sum3/1
  v_t/1 -> Sum3/2
  Sum3/1 -> Product/2
  Product/1 -> Sum4/1
  v_ly/1 -> Product1/2
  Product1/1 -> Sum4/2
  Sum4/1 -> Divide/2
  Divide/1 -> dl_dt/1
  Atan2/1 -> Derivative/1, theta_l/1
  Derivative/1 -> w_l/1

== system modelo_nioc_obs/Subsistema físico/Field Weaking Izaje ==
  w_hm : Inport
  Abs : Abs  SaturateOnIntegerOverflow=off
  Constant : Constant  Value=w_hm_rated
  Divide : Product  Inputs=*/
  Gain : Gain  Gain=T_hmMax
  Max : MinMax  Function=max  Inputs=2
  Square : Math  Operator=square
  T_hm_max : Outport
  wires:
  w_hm/1 -> Abs/1
  Constant/1 -> Divide/1, Max/2
  Divide/1 -> Square/1
  Square/1 -> Gain/1
  Gain/1 -> T_hm_max/1
  Abs/1 -> Max/1
  Max/1 -> Divide/2

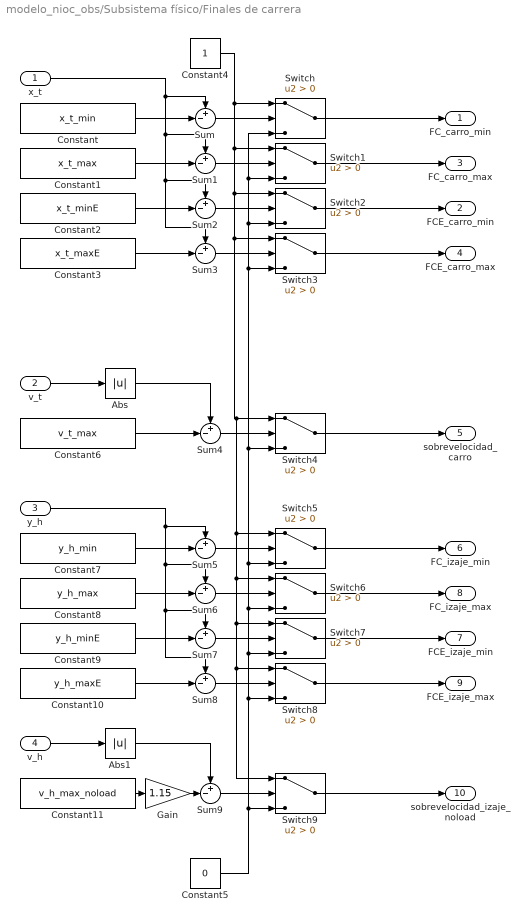
== system modelo_nioc_obs/Subsistema físico/Finales de carrera ==
  x_t : Inport
  v_t : Inport  Port=2
  y_h : Inport  Port=3
  v_h : Inport  Port=4
  Abs : Abs  SaturateOnIntegerOverflow=off
  Abs1 : Abs  SaturateOnIntegerOverflow=off
  Constant : Constant  Value=x_t_min
  Constant1 : Constant  Value=x_t_max
  Constant10 : Constant  Value=y_h_maxE
  Constant11 : Constant  Value=v_h_max_noload
  Constant2 : Constant  Value=x_t_minE
  Constant3 : Constant  Value=x_t_maxE
  Constant4 : Constant
  Constant5 : Constant  Value=0
  Constant6 : Constant  Value=v_t_max
  Constant7 : Constant  Value=y_h_min
  Constant8 : Constant  Value=y_h_max
  Constant9 : Constant  Value=y_h_minE
  Gain : Gain  Gain=1.15
  Sum{,1..9} (10 alike) : Sum  Inputs=+-|
  Switch{,1..9} (10 alike) : Switch  Criteria=u2 > Threshold  SaturateOnIntegerOverflow=off  InputSameDT=off
  FC_carro_min : Outport
  FCE_carro_min : Outport  Port=2
  FC_carro_max : Outport  Port=3
  FCE_carro_max : Outport  Port=4
  sobrevelocidad_carro : Outport  Port=5
  FC_izaje_min : Outport  Port=6
  FCE_izaje_min : Outport  Port=7
  FC_izaje_max : Outport  Port=8
  FCE_izaje_max : Outport  Port=9
  sobrevelocidad_izaje_noload : Outport  Port=10
  wires:
  Constant/1 -> Sum/2
  Constant1/1 -> Sum1/2
  Constant2/1 -> Sum2/2
  Constant3/1 -> Sum3/2
  x_t/1 -> Sum/1, Sum1/1, Sum2/1, Sum3/1
  Sum/1 -> Switch/2
  Constant4/1 -> Switch2/1, Switch9/1, Switch8/1, Switch7/1, Switch6/1, Switch5/1, Switch4/1, Switch3/1, Switch1/1, Switch/1
  Sum1/1 -> Switch1/2
  Sum2/1 -> Switch2/2
  Sum3/1 -> Switch3/2
  Switch/1 -> FC_carro_min/1
  Switch1/1 -> FC_carro_max/1
  Switch2/1 -> FCE_carro_min/1
  Switch3/1 -> FCE_carro_max/1
  v_t/1 -> Abs/1
  Constant6/1 -> Sum4/2
  Sum4/1 -> Switch4/2
  Abs/1 -> Sum4/1
  Switch4/1 -> sobrevelocidad_carro/1
  Switch7/1 -> FCE_izaje_min/1
  Switch6/1 -> FC_izaje_max/1
  y_h/1 -> Sum5/1, Sum6/1, Sum7/1, Sum8/1
  Sum7/1 -> Switch7/2
  Switch5/1 -> FC_izaje_min/1
  Constant7/1 -> Sum5/2
  Constant10/1 -> Sum8/2
  Constant9/1 -> Sum7/2
  Sum6/1 -> Switch6/2
  Constant8/1 -> Sum6/2
  Sum8/1 -> Switch8/2
  Constant5/1 -> Switch9/3, Switch8/3, Switch6/3, Switch5/3, Switch1/3, Switch/3, Switch2/3, Switch3/3, Switch4/3, Switch7/3
  Switch8/1 -> FCE_izaje_max/1
  Sum5/1 -> Switch5/2
  Constant11/1 -> Gain/1
  v_h/1 -> Abs1/1
  Abs1/1 -> Sum9/1
  Sum9/1 -> Switch9/2
  Switch9/1 -> sobrevelocidad_izaje_noload/1
  Gain/1 -> Sum9/2

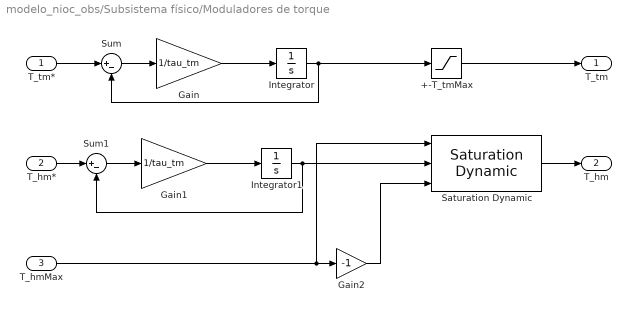
== system modelo_nioc_obs/Subsistema físico/Moduladores de torque ==
  T_tm* : Inport
  T_hm* : Inport  Port=2
  T_hmMax : Inport  Port=3
  +-T_tmMax : Saturate  UpperLimit=+T_tmMax  LowerLimit=-T_tmMax
  Gain : Gain  Gain=1/tau_tm
  Gain1 : Gain  Gain=1/tau_tm
  Gain2 : Gain  Gain=-1
  Integrator : Integrator
  Integrator1 : Integrator
  Saturation Dynamic : simulink/Discontinuities/Saturation Dynamic  OutMin=[]  OutMax=[]  OutDataTypeStr=Inherit: Same as second input  OutDataType=fixdt(1, 16)  OutScaling=2^-10  DoSatur=off
  Sum : Sum  Inputs=|+-
  Sum1 : Sum  Inputs=|+-
  T_tm : Outport
  T_hm : Outport  Port=2
  wires:
  +-T_tmMax/1 -> T_tm/1
  Gain/1 -> Integrator/1
  Integrator/1 -> Sum/2, +-T_tmMax/1
  T_tm*/1 -> Sum/1
  Sum/1 -> Gain/1
  Gain1/1 -> Integrator1/1
  Sum1/1 -> Gain1/1
  Integrator1/1 -> Sum1/2, Saturation Dynamic/2
  T_hm*/1 -> Sum1/1
  Saturation Dynamic/1 -> T_hm/1
  T_hmMax/1 -> Gain2/1, Saturation Dynamic/1
  Gain2/1 -> Saturation Dynamic/3

== system modelo_nioc_obs/Subsistema físico/Accionamiento Carro/Subsystem ==
  BRK_t : Inport
  w_tm : Inport  Port=2
  +-T_tbmax : Saturate  UpperLimit=T_tbMax  LowerLimit=-T_tbMax
  Constant : Constant  Value=0
  Gain : Gain  Gain=-b_tb
  Gain1 : Gain  Gain=-T_tbMax
  Switch : Switch  Criteria=u2 > Threshold  SaturateOnIntegerOverflow=off  InputSameDT=off
  Tanh : Trigonometry  Operator=tanh
  T_tb : Outport
  wires:
  BRK_t/1 -> Switch/2
  Constant/1 -> Switch/1
  Gain/1 -> Tanh/1
  w_tm/1 -> Gain/1
  Switch/1 -> +-T_tbmax/1
  +-T_tbmax/1 -> T_tb/1
  Tanh/1 -> Gain1/1
  Gain1/1 -> Switch/3

== system modelo_nioc_obs/Subsistema físico/Accionamiento Izaje/Freno de operación ==
  BRK_h : Inport
  w_hm : Inport  Port=2
  +-T_hbmax : Saturate  UpperLimit=T_hbMax  LowerLimit=-T_hbMax
  Constant : Constant  Value=0
  Gain : Gain  Gain=b_hb
  Gain1 : Gain  Gain=-T_hbMax
  Switch : Switch  Criteria=u2 > Threshold  SaturateOnIntegerOverflow=off  InputSameDT=off
  Tanh : Trigonometry  Operator=tanh
  T_hb : Outport
  wires:
  BRK_h/1 -> Switch/2
  Constant/1 -> Switch/1
  Gain/1 -> Tanh/1
  w_hm/1 -> Gain/1
  Switch/1 -> +-T_hbmax/1
  +-T_hbmax/1 -> T_hb/1
  Tanh/1 -> Gain1/1
  Gain1/1 -> Switch/3

== system modelo_nioc_obs/Subsistema físico/Accionamiento Izaje/Freno de operación1 ==
  BRK_hE : Inport
  w_hd : Inport  Port=2
  +-T_hEbmax : Saturate  UpperLimit=T_hEbMax  LowerLimit=-T_hEbMax
  Constant : Constant  Value=0
  Gain : Gain  Gain=b_hd
  Gain1 : Gain  Gain=-T_hEbMax
  Switch : Switch  Criteria=u2 > Threshold  SaturateOnIntegerOverflow=off  InputSameDT=off
  Tanh : Trigonometry  Operator=tanh
  T_hEb : Outport
  wires:
  BRK_hE/1 -> Switch/2
  Constant/1 -> Switch/1
  Gain/1 -> Tanh/1
  w_hd/1 -> Gain/1
  Switch/1 -> +-T_hEbmax/1
  +-T_hEbmax/1 -> T_hEb/1
  Tanh/1 -> Gain1/1
  Gain1/1 -> Switch/3

== system modelo_nioc_obs/Subsistema físico/Cable izaje/Calculo K_hw ==
  l_h : Inport
  Constant : Constant  Value=110
  Constant1 : Constant  Value=k_wu
  Divide : Product  Inputs=*/
  Gain : Gain  Gain=2
  Sum : Sum  Inputs=|++
  K_hw : Outport
  wires:
  l_h/1 -> Gain/1
  Gain/1 -> Sum/1
  Constant/1 -> Sum/2
  Sum/1 -> Divide/2
  Constant1/1 -> Divide/1
  Divide/1 -> K_hw/1

== system modelo_nioc_obs/Subsistema físico/Cable izaje/Calculo b_hw ==
  l_h : Inport
  Constant : Constant  Value=110
  Gain : Gain  Gain=2
  Gain1 : Gain  Gain=b_wu
  Sum : Sum  Inputs=|++
  b_hw : Outport
  wires:
  l_h/1 -> Gain/1
  Gain/1 -> Sum/1
  Constant/1 -> Sum/2
  Sum/1 -> Gain1/1
  Gain1/1 -> b_hw/1

== system modelo_nioc_obs/Subsistema físico/Carga/F_cx ==
  h_c : Inport
  y_c0 : Inport  Port=2
  y_l : Inport  Port=3
  v_lx : Inport  Port=4
  Constant : Constant  Value=0
  Gain : Gain  Gain=-b_cx
  Sum : Sum  Inputs=|+-
  Sum1 : Sum  Inputs=|-+
  Switch : Switch  Criteria=u2 > Threshold  SaturateOnIntegerOverflow=off  InputSameDT=off
  F_cx : Outport
  wires:
  y_l/1 -> Sum/1
  h_c/1 -> Sum/2
  Sum/1 -> Sum1/1
  y_c0/1 -> Sum1/2
  Sum1/1 -> Switch/2
  Constant/1 -> Switch/3
  v_lx/1 -> Gain/1
  Gain/1 -> Switch/1
  Switch/1 -> F_cx/1

== system modelo_nioc_obs/Subsistema físico/Carga/F_cy ==
  y_l : Inport
  v_ly : Inport  Port=2
  h_c : Inport  Port=3
  y_c0 : Inport  Port=4
  Constant1 : Constant  Value=0
  Gain : Gain  Gain=K_cy
  Gain1 : Gain  Gain=b_cy
  Sum : Sum  Inputs=|+-
  Sum1 : Sum  Inputs=|-+
  Sum2 : Sum  Inputs=|+-
  Sum3 : Sum  Inputs=|-+
  switch : Switch  Criteria=u2 > Threshold  SaturateOnIntegerOverflow=off  InputSameDT=off
  F_cy : Outport
  wires:
  switch/1 -> F_cy/1
  Sum2/1 -> switch/1
  Constant1/1 -> switch/3
  Sum/1 -> Sum3/1, Sum1/1
  y_l/1 -> Sum/1
  h_c/1 -> Sum/2
  y_c0/1 -> Sum3/2, Sum1/2
  Sum1/1 -> Gain/1
  Gain/1 -> Sum2/1
  v_ly/1 -> Gain1/1
  Gain1/1 -> Sum2/2
  Sum3/1 -> switch/2

== matlab function modelo_nioc_obs/Generador Trayectoria ==
  data: t input; t_inicio input; x_t_star output; x_inicial input; x_final input; v_t_star output; a_t_star output
function [x_t_star, v_t_star, a_t_star] = generador_trayectoria(t, t_inicio, x_inicial, x_final)
    % ---------------------------------------------------------------------
    % LIMITES OPERATIVOS (Sección 3.3) - PERFIL EN "S" (Jerk Limitado)
    % ---------------------------------------------------------------------
    v_max_limite = 4.0; % [m/s]
    a_max_limite = 0.8; % [m/s^2]
    
    % ESCUDO DE ESPERA
    if t < t_inicio
        x_t_star = x_inicial;
        v_t_star = 0;
        a_t_star = 0;
        return;
    end
    
    t_eff = t - t_inicio;
    D = abs(x_final - x_inicial);
    dir = sign(x_final - x_inicial);
    
    if D == 0
        x_t_star = x_inicial;
        v_t_star = 0;
        a_t_star = 0;
        return;
    end
    
    % ---------------------------------------------------------------------
    % CALCULO DEL PERFIL SENOIDAL (S-Curve)
    % ---------------------------------------------------------------------
    % Tiempo y distancia teórica para aceleración senoidal completa
    t_a = (pi * v_max_limite) / (2 * a_max_limite);
    d_a = (v_max_limite * t_a) / 2;
    
    if 2 * d_a >= D
        % El trayecto es corto: No llega a velocidad crucero (Perfil campana)
        v_pico = sqrt((2 * a_max_limite * D) / pi);
        t_a = (pi * v_pico) / (2 * a_max_limite);
        t_crucero = 0;
        v_crucero = v_pico;
        d_crucero = 0;
        d_a = D / 2;
    else
        % El trayecto es largo: Perfil en "S" con tramo de crucero plano
        v_crucero = v_max_limite;
        d_crucero = D - 2 * d_a;
        t_crucero = d_crucero / v_crucero;
    end
    
    t_total = 2 * t_a + t_crucero;
    
    % ---------------------------------------------------------------------
    % ECUACIONES CINEMÁTICAS INTEGRADAS (Onda Seno)
    % ---------------------------------------------------------------------
    if t_eff < t_a
        % Fase 1: Aceleración Suave (Onda Seno)
        a_t_star = a_max_limite * sin(pi * t_eff / t_a) * dir;
        v_t_star = (a_max_limite * t_a / pi) * (1 - cos(pi * t_eff / t_a)) * dir;
        x_t_star = x_inicial + ((a_max_limite * t_a / pi) * (t_eff - (t_a / pi) * sin(pi * t_eff / t_a))) * dir;
        
    elseif t_eff < (t_a + t_crucero)
        % Fase 2: Velocidad Constante (Crucero)
        t_fase2 = t_eff - t_a;
        a_t_star = 0;
        v_t_star = v_crucero * dir;
        x_t_star = x_inicial + d_a * dir + v_crucero * t_fase2 * dir;
        
    elseif t_eff < t_total
        % Fase 3: Desaceleración Suave (Onda Seno invertida)
        t_fase3 = t_eff - (t_a + t_crucero);
        a_t_star = -a_max_limite * sin(pi * t_fase3 / t_a) * dir;
        v_t_star = (v_crucero - (a_max_limite * t_a / pi) * (1 - cos(pi * t_fase3 / t_a))) * dir;
        x_t_star = x_inicial + (d_a + d_crucero) * dir + (v_crucero * t_fase3 - (a_max_limite * t_a / pi) * (t_fase3 - (t_a / pi) * sin(pi * t_fase3 / t_a))) * dir;
        
    else
        % Fase 4: Destino
        x_t_star = x_final;
        v_t_star = 0;
        a_t_star = 0;
    end
end

== matlab function modelo_nioc_obs/Controlador de Balanceo/MATLAB Function ==
  data: theta_l input; a_PD output; w_l input; l input; dl_dt input; g input
function a_PD = controlador_balanceo(theta_l, w_l, l, dl_dt, g)
    % 1. Escudos de seguridad
    if l < 0.1
        l_seguro = 0.1;
    else
        l_seguro = l;
    end

    theta_max = 80 * (pi/180);
    if theta_l > theta_max
        theta_math = theta_max;
    elseif theta_l < -theta_max
        theta_math = -theta_max;
    else
        theta_math = theta_l;
    end

    if abs(theta_math) < 1e-4
        sinc_theta = 1;
    else
        sinc_theta = sin(theta_math) / theta_math;
    end

    % 2. EL CORTACORRIENTE (ZONA MUERTA)
    % Apaga nuestra corrección si el péndulo ya casi no se mueve
    if abs(theta_math) < 0.005 && abs(w_l) < 0.01
        a_PD = 0;
        return; 
    end

    % 3. Frecuencia natural dinámica (Opción 1)
    w_o = 2*sqrt(g / l_seguro);

    % 4. Fórmulas LPV
    K_po = (g * sinc_theta - (w_o^2) * l_seguro) / cos(theta_math);
    K_do = (2 * dl_dt - 2 * w_o * l_seguro) / cos(theta_math);

    % 5. Salida de control
    a_PD = - K_po * theta_l - K_do * w_l;
end

== matlab function modelo_nioc_obs/MATLAB Function1 ==
  data: t input; l_h_star output; t_inicio input; l_inicial input; l_final input; masa_total input; dl_h_star output; ddl_h_star output
function [l_h_star, dl_h_star, ddl_h_star] = generador_trayectoria_izaje(t, t_inicio, l_inicial, l_final, masa_total)
    % ---------------------------------------------------------------------
    % CONSTANTES FISICAS Y OPERATIVAS DE IZAJE
    % ---------------------------------------------------------------------
    g = 9.80665;               
    P_const = 956150;          
    v_max_absoluta = 3.0;      
    a_max_limite = 0.75;       
    
    % Operación a potencia constante según carga actual
    v_potencia = P_const / (masa_total * g);
    v_max_limite = min(v_max_absoluta, v_potencia);
    
    if t < t_inicio
        l_h_star = l_inicial;
        dl_h_star = 0;
        ddl_h_star = 0;
        return;
    end
    
    t_eff = t - t_inicio;
    D = abs(l_final - l_inicial);
    dir = sign(l_final - l_inicial); 
    
    if D == 0
        l_h_star = l_inicial;
        dl_h_star = 0;
        ddl_h_star = 0;
        return;
    end
    
    % ---------------------------------------------------------------------
    % CALCULO DEL PERFIL CINEMATICO (Curva S con Jerk continuo: 1 - cos)
    % ---------------------------------------------------------------------
    % Tiempo para alcanzar la velocidad máxima con este perfil
    t_a = 2 * v_max_limite / a_max_limite;
    d_a = v_max_limite * t_a / 2;
    
    if 2 * d_a >= D
        % Perfil sin crucero (Triangular ultra-suavizado)
        v_pico = sqrt((D * a_max_limite) / 2);
        t_a = 2 * v_pico / a_max_limite;
        t_crucero = 0;
        v_crucero = v_pico;
        d_crucero = 0;
        d_a = D / 2;
    else
        % Perfil Trapezoidal ultra-suavizado
        v_crucero = v_max_limite;
        d_crucero = D - 2 * d_a;
        t_crucero = d_crucero / v_crucero;
    end
    
    t_total = 2 * t_a + t_crucero;
    
    % ---------------------------------------------------------------------
    % EVALUACION INSTANTANEA
    % ---------------------------------------------------------------------
    if t_eff < t_a
        % Fase 1: Aceleración Suave (Perfil campana 1-cos)
        ddl_h_star = (a_max_limite / 2) * (1 - cos(2 * pi * t_eff / t_a)) * dir;
        dl_h_star = (a_max_limite / 2) * (t_eff - (t_a / (2 * pi)) * sin(2 * pi * t_eff / t_a)) * dir;
        l_h_star = l_inicial + (a_max_limite / 2) * ((t_eff^2 / 2) + (t_a^2 / (4 * pi^2)) * (cos(2 * pi * t_eff / t_a) - 1)) * dir;
        
    elseif t_eff < (t_a + t_crucero)
        % Fase 2: Velocidad Constante de Crucero
        t_fase2 = t_eff - t_a;
        ddl_h_star = 0;
        dl_h_star = v_crucero * dir;
        l_h_star = l_inicial + d_a * dir + v_crucero * t_fase2 * dir;
        
    elseif t_eff < t_total
        % Fase 3: Desaceleración Suave (Campana invertida 1-cos)
        t_fase3 = t_eff - (t_a + t_crucero);
        ddl_h_star = -(a_max_limite / 2) * (1 - cos(2 * pi * t_fase3 / t_a)) * dir;
        dl_h_star = (v_crucero - (a_max_limite / 2) * (t_fase3 - (t_a / (2 * pi)) * sin(2 * pi * t_fase3 / t_a))) * dir;
        
        d_recorrida_fase3 = v_crucero * t_fase3 - (a_max_limite / 2) * ((t_fase3^2 / 2) + (t_a^2 / (4 * pi^2)) * (cos(2 * pi * t_fase3 / t_a) - 1));
        l_h_star = l_inicial + (d_a + d_crucero + d_recorrida_fase3) * dir;
        
    else
        % Fase 4: Posición final alcanzada
        l_h_star = l_final;
        dl_h_star = 0;
        ddl_h_star = 0;
    end
end

== matlab function modelo_nioc_obs/Subsistema físico/MATLAB Function ==
  data: x_t_min input; y_c0_contacto output; x_t_max input; Y_sb input; W_c input; y_h_min input; H_c input; x_lidar_offset input; x_l input; TLK input; y_c0_lidar output
function [y_c0_contacto, y_c0_lidar] = perfil_suelo(x_t_min, x_t_max, Y_sb, W_c, y_h_min, H_c, x_lidar_offset, x_l, TLK)

persistent n_containers x_grid tlk_prev

%% Inicialización de perfil

if isempty(n_containers)
    x_grid       = x_t_min : W_c : x_t_max;
    n_containers = zeros(1, length(x_grid));
    tlk_prev     = 0;
end

%% Índice más cercano a x_l

[~, idx] = min(abs(x_grid - x_l));

%% Extracción y depósito de contenedores

flanco_bajada = (tlk_prev == 1) && (TLK == 0);
flanco_subida = (tlk_prev == 0) && (TLK == 1);

if flanco_bajada
    n_containers(idx) = n_containers(idx) + 1;
elseif flanco_subida
    n_containers(idx) = max(0, n_containers(idx) - 1);
end

tlk_prev = TLK;

%% Altura fija según zona
if x_l < -W_c/2
    y_fijo = 0;
elseif x_l >= -W_c/2 && x_l <= W_c/2
    y_fijo = Y_sb;
else
    y_fijo = y_h_min;
end

%% Altura total
y_c0_contacto = y_fijo + n_containers(idx) * H_c;

%% Lectura de lidar
x_laser = x_l + x_lidar_offset; % Definimos la posición exacta del láser
[~, idx_lidar] = min(abs(x_grid - x_laser));

% Ahora evaluamos las zonas usando la visión del láser, no de la carga
if x_laser < -W_c/2
    y_fijo_lidar = 0;
elseif x_laser >= -W_c/2 && x_laser <= W_c/2
    y_fijo_lidar = Y_sb;
else
    y_fijo_lidar = y_h_min;
end

y_c0_lidar = y_fijo_lidar + n_containers(idx_lidar) * H_c;
